simulink model "SegwayModelLinearized02017"  (R2018b)
settings: Solver=VariableStepAuto  StartTime=0.0  StopTime=10.0  RelTol=1e-3
undefined symbols (not defined in the file): A, B, F, T, X0lin0
settings Model: Creator=Huynh  LastModifiedBy=Huynh
settings DataIOCC: ReturnWorkspaceOutputs=on

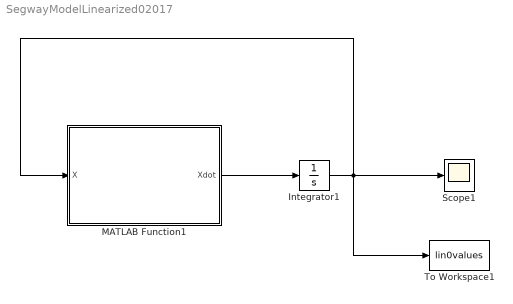
== system SegwayModelLinearized02017 ==
  Integrator1 : Integrator  InitialCondition=X0lin0
  MATLAB Function1 : MATLAB Function  TreatAsAtomicUnit=on
  Scope1 : Scope
  To Workspace1 : ToWorkspace  VariableName=lin0values  SampleTime=-1
  wires:
  MATLAB Function1/1(Xdot) -> Integrator1/1
  Integrator1/1 -> MATLAB Function1/1(X), To Workspace1/1, Scope1/1

== matlab function SegwayModelLinearized02017/MATLAB Function1 ==
  data: X input; Xdot output; A parameter; B parameter; T parameter; F parameter
function Xdot = LinearZeroSegway(X, A, B, T, F)
u = [T; F];
Xdot = A * X + B * u;
end
